simulink model "MOSSE_HDL_code_gen_final"  (Simulink 8.2)
settings: Solver=FixedStepDiscrete  SolverMode=SingleTasking  StartTime=0.0  StopTime=20*640*360  RelTol=1e-3
InitFcn:
  | %% DSPBuilder Start
  | alt_dspbuilder_update_model(bdroot)
  | %% DSPBuilder End
  | param
StopFcn:
  | % r = rcount.Data(:,:);
  | % w = wcount.Data(:,:);
  | % d = dout.Data(:,:);
  | % ir = read.Data(:,:);
  | % iw = write.Data(:,:);
  | % z = double([ir iw d r w]');
  | %logic_analyzer
values from neighbouring files (symbols this model uses):
  Gau = [4035 -3983 3832 -3589 3269 -2890 2472 -2039 1612 -1211 854 -553 ... (4096 elements, 1x4096)]    [Gauss_coeff.mat]    (also in param.m = reshape(conj(Gau'), 1, 4096))
undefined symbols (not defined in the file or in its folder): jet, psr, source_1, source_2, State_Machine, State_Transition_Table1, window_hann
libraries: allblocks_alteradspbuilder2 x182, hdldemolib x2, dspsigattribs x2, dspmtrx3 x2, visionsinks x1, visiontextngfix x1, dspvision x1
(part 2 of 3)

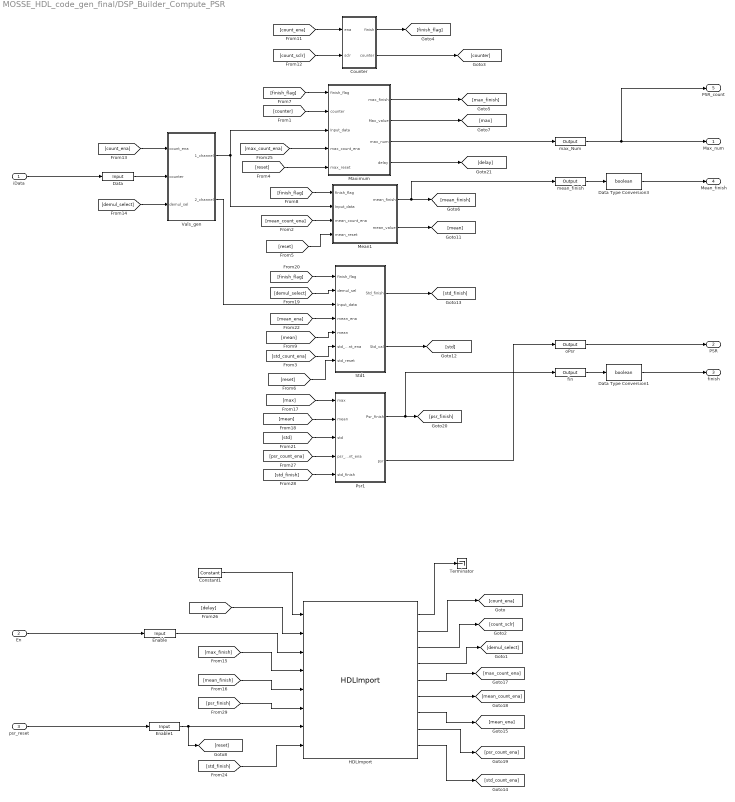
== system MOSSE_HDL_code_gen_final/DSP_Builder_Compute_PSR ==
  iData : Inport
  En : Inport  Port=2
  psr_reset : Inport  Port=3
  Constant1 : allblocks_alteradspbuilder2/Constant  mask_cst=1  BusType=Single Bit  bwl=8  bwr=0  roundMode=Truncate  satMode=Wrap  SpecifyClock=off  allowFloatingPointOverride=on  logOutputs=off  logFile=d:\Project\AutoTracking\model\MOSSE_work\MOSSE_model\MOSSE_Final_models\tb_MOSSE_HDL_final\MOSSE%5FHDL%5Ffinal_DSP%5FBuilder%5FCompute%5FPSR_Constant1.fixedpointlog
  Counter : Subsystem
  Data : allblocks_alteradspbuilder2/Input  iofile=d:\Project\AutoTracking\model\MOSSE_work\MOSSE_model\MOSSE_Final_models\tb_MOSSE_HDL_final\MOSSE%5FHDL%5Ffinal_DSP%5FBuilder%5FCompute%5FPSR_Data.salt  BusType=Signed Integer  bwl=16  bwr=0  SpecifyClock=off  PORTTYPE=Input  externalType=Inferred  allowFloatingPointOverride=on  logOutputs=off
  Data Type Conversion1 : DataTypeConversion  OutDataTypeStr=boolean
  Data Type Conversion3 : DataTypeConversion  OutDataTypeStr=boolean
  Enable : allblocks_alteradspbuilder2/Input  iofile=d:\Project\AutoTracking\model\MOSSE_work\MOSSE_model\MOSSE_Final_models\tb_MOSSE_HDL_final\MOSSE%5FHDL%5Ffinal_DSP%5FBuilder%5FCompute%5FPSR_Enable.salt  BusType=Single Bit  bwl=16  bwr=0  SpecifyClock=off  PORTTYPE=Input  externalType=Inferred  allowFloatingPointOverride=on  logOutputs=off
  Enable1 : allblocks_alteradspbuilder2/Input  iofile=d:\Project\AutoTracking\model\MOSSE_work\MOSSE_model\MOSSE_Final_models\tb_MOSSE_HDL_final\MOSSE%5FHDL%5Ffinal_DSP%5FBuilder%5FCompute%5FPSR_Enable1.salt  BusType=Single Bit  bwl=16  bwr=0  SpecifyClock=off  PORTTYPE=Input  externalType=Inferred  allowFloatingPointOverride=on  logOutputs=off
  HDLImport : allblocks_alteradspbuilder2/HDLImport  entityName=State_Machine_import  inNames=clk_enable delay enable_in max_finish mean_finish psr_finish reset std_finish  inBwls=1 1 1 1 1 1 1 1  inBwrs="0  0  0  0  0  0  0  0"  inTypes=b b b b b b b b  inDelayed="0  0  0  0  0  0  0  0"  outNames=ce_out count_ena count_sclr demul_select max_count_ena mean_count_ena mean_ena psr_count_ena std_count_ena  outBwls=1 1 1 1 1 1 1 1 1  outBwrs="0  0  0  0  0  0  0  0  0"  outTypes=b b b b b b b b b  xmlmapfile=C:\altera\13.0\quartus\dsp_builder\lib\SimgenCMap.xml  vofile=DSPBuilder_MOSSE_HDL_final_import\State_Machine.vo  src_file=psr\State_Machine.v;psr\State_Transition_Table1.v;  TopLevelName=State_Machine  UseQPF=0  n_input_port=8  n_output_port=9  array_clocks=clk  use_systemC_model=off  is_megacore=off  use_dynamic_feedthrough_data=off  use_alphabetical_port_ordering=on  allowFloatingPointOverride=off
  Maximum : Subsystem
  Mean1 : Subsystem
  Psr1 : Subsystem
  Std1 : Subsystem
  Terminator : Terminator
  Vals_gen : Subsystem
  fin : allblocks_alteradspbuilder2/Output  iofile=d:\Project\AutoTracking\model\MOSSE_work\MOSSE_model\MOSSE_Final_models\tb_MOSSE_HDL_final\MOSSE%5FHDL%5Ffinal_DSP%5FBuilder%5FCompute%5FPSR_fin.capture  BusType=Single Bit  bwl=32  bwr=0  externalType=Simulink Fixed Point Type  PORTTYPE=Output  allowFloatingPointOverride=on  logOutputs=off
  max_Num : allblocks_alteradspbuilder2/Output  iofile=d:\Project\AutoTracking\model\MOSSE_work\MOSSE_model\MOSSE_Final_models\tb_MOSSE_HDL_final\MOSSE%5FHDL%5Ffinal_DSP%5FBuilder%5FCompute%5FPSR_max%5FNum.capture  BusType=Signed Integer  bwl=16  bwr=0  externalType=Simulink Fixed Point Type  PORTTYPE=Output  allowFloatingPointOverride=on  logOutputs=off
  mean_finish : allblocks_alteradspbuilder2/Output  iofile=d:\Project\AutoTracking\model\MOSSE_work\MOSSE_model\MOSSE_Final_models\tb_MOSSE_HDL_final\MOSSE%5FHDL%5Ffinal_DSP%5FBuilder%5FCompute%5FPSR_mean%5Ffinish.capture  BusType=Single Bit  bwl=16  bwr=0  externalType=Simulink Fixed Point Type  PORTTYPE=Output  allowFloatingPointOverride=on  logOutputs=off
  oPsr : allblocks_alteradspbuilder2/Output  iofile=d:\Project\AutoTracking\model\MOSSE_work\MOSSE_model\MOSSE_Final_models\tb_MOSSE_HDL_final\MOSSE%5FHDL%5Ffinal_DSP%5FBuilder%5FCompute%5FPSR_oPsr.capture  BusType=Signed Integer  bwl=32  bwr=0  externalType=Simulink Fixed Point Type  PORTTYPE=Output  allowFloatingPointOverride=on  logOutputs=off
  Max_num : Outport
  PSR : Outport  Port=2
  finish : Outport  Port=3
  Mean_finish : Outport  Port=4
  PSR_count : Outport  Port=5
  wires:
  [demul_select] -> Std1/2(demul_sel)
  Data/1 -> Vals_gen/2(counter)
  [demul_select] -> Vals_gen/3(demul_sel)
  Vals_gen/2(2_channel) -> Std1/3(Input_data)
  [finish_flag] -> Std1/1(finish_flag)
  Std1/1(Std_finish) -> [std_finish]
  Mean1/2(mean_value) -> [mean]
  max_Num/1 -> PSR_count/1, Max_num/1
  Maximum/2(Max_value) -> [max]
  [mean] -> Std1/5(mean)
  [mean_ena] -> Std1/4(mean_ena)
  [max] -> Psr1/1(max)
  Maximum/4(delay) -> [delay]
  HDLImport/1 -> Terminator/1
  Constant1/1 -> HDLImport/1
  [psr_finish] -> HDLImport/6
  [std_finish] -> HDLImport/8
  [mean_finish] -> HDLImport/5
  [max_finish] -> HDLImport/4
  [delay] -> HDLImport/2
  Mean1/1(mean_finish) -> mean_finish/1, [mean_finish]
  oPsr/1 -> PSR/1
  [count_ena] -> Vals_gen/1(count_ena)
  Psr1/1(Psr_finish) -> fin/1, [psr_finish]
  Vals_gen/1(1_channel) -> Maximum/3(Input_data), Mean1/2(Input_data)
  [mean_count_ena] -> Mean1/3(mean_count_ena)
  Counter/1(finish) -> [finish_flag]
  Maximum/1(max_finish) -> [max_finish]
  [counter] -> Maximum/2(counter)
  [finish_flag] -> Maximum/1(finish_flag)
  [finish_flag] -> Mean1/1(finish_flag)
  [count_ena] -> Counter/1(ena)
  [count_sclr] -> Counter/2(sclr)
  [std_finish] -> Psr1/5(std_finish)
  Psr1/2(psr) -> oPsr/1
  [mean] -> Psr1/2(mean)
  [std] -> Psr1/3(std)
  Std1/2(Std_val) -> [std]
  [std_count_ena] -> Std1/6(std_count_ena)
  [psr_count_ena] -> Psr1/4(psr_count_ena)
  [max_count_ena] -> Maximum/4(max_count_ena)
  HDLImport/3 -> [count_sclr]
  HDLImport/2 -> [count_ena]
  HDLImport/6 -> [mean_count_ena]
  Enable/1 -> HDLImport/3
  HDLImport/4 -> [demul_select]
  HDLImport/5 -> [max_count_ena]
  HDLImport/7 -> [mean_ena]
  HDLImport/8 -> [psr_count_ena]
  HDLImport/9 -> [std_count_ena]
  Counter/2(counter) -> [counter]
  En/1 -> Enable/1
  iData/1 -> Data/1
  psr_reset/1 -> Enable1/1
  Enable1/1 -> [reset], HDLImport/7
  mean_finish/1 -> Data Type Conversion3/1
  fin/1 -> Data Type Conversion1/1
  Data Type Conversion1/1 -> finish/1
  Data Type Conversion3/1 -> Mean_finish/1
  [reset] -> Maximum/5(max_reset)
  [reset] -> Mean1/4(mean_reset)
  [reset] -> Std1/7(std_reset)
  Maximum/3(max_num) -> max_Num/1

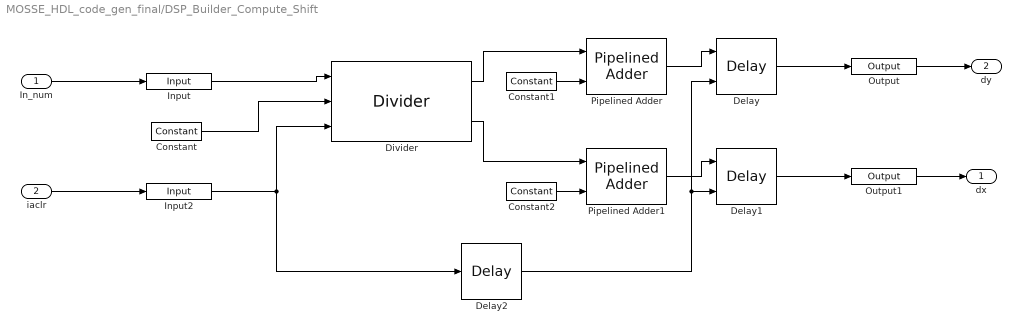
== system MOSSE_HDL_code_gen_final/DSP_Builder_Compute_Shift ==
  In_num : Inport
  iaclr : Inport  Port=2
  Constant : allblocks_alteradspbuilder2/Constant  mask_cst=64  BusType=Unsigned Integer  bwl=8  bwr=0  roundMode=Truncate  satMode=Wrap  SpecifyClock=off  allowFloatingPointOverride=on  logOutputs=off  logFile=C:\Workspace\Autotracking\MOSSE_model\tb_MOSSE_HDL_final\MOSSE%5FHDL%5Ffinal_DSP%5FBuilder%5FCompute%5FShift_Constant.fixedpointlog
  Constant1 : allblocks_alteradspbuilder2/Constant  mask_cst=31  BusType=Signed Integer  bwl=8  bwr=0  roundMode=Truncate  satMode=Wrap  SpecifyClock=off  allowFloatingPointOverride=on  logOutputs=off  logFile=C:\Workspace\Autotracking\MOSSE_model\tb_MOSSE_HDL_final\MOSSE%5FHDL%5Ffinal_DSP%5FBuilder%5FCompute%5FShift_Constant1.fixedpointlog
  Constant2 : allblocks_alteradspbuilder2/Constant  mask_cst=32  BusType=Signed Integer  bwl=8  bwr=0  roundMode=Truncate  satMode=Wrap  SpecifyClock=off  allowFloatingPointOverride=on  logOutputs=off  logFile=C:\Workspace\Autotracking\MOSSE_model\tb_MOSSE_HDL_final\MOSSE%5FHDL%5Ffinal_DSP%5FBuilder%5FCompute%5FShift_Constant2.fixedpointlog
  Delay : allblocks_alteradspbuilder2/Delay  pipeline=1  pipeline_display=1  ClockPhase=1  use_ena=off  use_sclr=on  allowFloatingPointOverride=on  logOutputs=off  logFile=C:\Workspace\Autotracking\MOSSE_model\tb_MOSSE_HDL_final\MOSSE%5FHDL%5Ffinal_DSP%5FBuilder%5FCompute%5FShift_Delay.fixedpointlog  use_init=off  reset_value=1
  Delay1 : allblocks_alteradspbuilder2/Delay  pipeline=1  pipeline_display=1  ClockPhase=1  use_ena=off  use_sclr=on  allowFloatingPointOverride=on  logOutputs=off  logFile=C:\Workspace\Autotracking\MOSSE_model\tb_MOSSE_HDL_final\MOSSE%5FHDL%5Ffinal_DSP%5FBuilder%5FCompute%5FShift_Delay1.fixedpointlog  use_init=off  reset_value=1
  Delay2 : allblocks_alteradspbuilder2/Delay  pipeline=1  pipeline_display=1  ClockPhase=1  use_ena=off  use_sclr=off  allowFloatingPointOverride=on  logOutputs=off  logFile=C:\Workspace\Autotracking\MOSSE_model\tb_MOSSE_HDL_final\MOSSE%5FHDL%5Ffinal_DSP%5FBuilder%5FCompute%5FShift_Delay2.fixedpointlog  use_init=off  reset_value=1
  Divider : allblocks_alteradspbuilder2/Divider  BusType=Unsigned Integer  bwl=12  bwr=0  pipeline=1  pipeline_display=1  use_ena=off  use_aclr=on
  Input : allblocks_alteradspbuilder2/Input  iofile=C:\Workspace\Autotracking\MOSSE_model\tb_MOSSE_HDL_final\MOSSE%5FHDL%5Ffinal_DSP%5FBuilder%5FCompute%5FShift_Input.salt  BusType=Unsigned Integer  bwl=12  bwr=0  SpecifyClock=off  PORTTYPE=Input  externalType=Inferred  allowFloatingPointOverride=on  logOutputs=off
  Input2 : allblocks_alteradspbuilder2/Input  iofile=C:\Workspace\Autotracking\MOSSE_model\tb_MOSSE_HDL_final\MOSSE%5FHDL%5Ffinal_DSP%5FBuilder%5FCompute%5FShift_Input2.salt  BusType=Single Bit  bwl=12  bwr=0  SpecifyClock=off  PORTTYPE=Input  externalType=Inferred  allowFloatingPointOverride=on  logOutputs=off
  Output : allblocks_alteradspbuilder2/Output  iofile=C:\Workspace\Autotracking\MOSSE_model\tb_MOSSE_HDL_final\MOSSE%5FHDL%5Ffinal_DSP%5FBuilder%5FCompute%5FShift_Output.capture  BusType=Signed Integer  bwl=8  bwr=0  externalType=Simulink Fixed Point Type  PORTTYPE=Output  allowFloatingPointOverride=on  logOutputs=off
  Output1 : allblocks_alteradspbuilder2/Output  iofile=C:\Workspace\Autotracking\MOSSE_model\tb_MOSSE_HDL_final\MOSSE%5FHDL%5Ffinal_DSP%5FBuilder%5FCompute%5FShift_Output1.capture  BusType=Signed Integer  bwl=8  bwr=0  externalType=Simulink Fixed Point Type  PORTTYPE=Output  allowFloatingPointOverride=on  logOutputs=off
  Pipelined Adder : allblocks_alteradspbuilder2/Pipelined Adder  BusType=Signed Integer  bwl=12  bwr=0  pipeline=0  pipeline_display=0  AddSubDirection=SUB  use_cin=off  use_ovl=off  use_addsub=off  use_ena=off  use_aclr=off  or_aclr_inputs=on
  Pipelined Adder1 : allblocks_alteradspbuilder2/Pipelined Adder  BusType=Signed Integer  bwl=12  bwr=0  pipeline=0  pipeline_display=0  AddSubDirection=SUB  use_cin=off  use_ovl=off  use_addsub=off  use_ena=off  use_aclr=off  or_aclr_inputs=on
  dx : Outport
  dy : Outport  Port=2
  wires:
  Input/1 -> Divider/1
  Constant/1 -> Divider/2
  In_num/1 -> Input/1
  Output1/1 -> dx/1
  Output/1 -> dy/1
  Divider/1 -> Pipelined Adder/1
  Constant2/1 -> Pipelined Adder1/2
  Pipelined Adder/1 -> Delay/1
  Delay/1 -> Output/1
  Pipelined Adder1/1 -> Delay1/1
  Delay1/1 -> Output1/1
  Divider/2 -> Pipelined Adder1/1
  iaclr/1 -> Input2/1
  Input2/1 -> Delay2/1, Divider/3
  Constant1/1 -> Pipelined Adder/2
  Delay2/1 -> Delay/2, Delay1/2

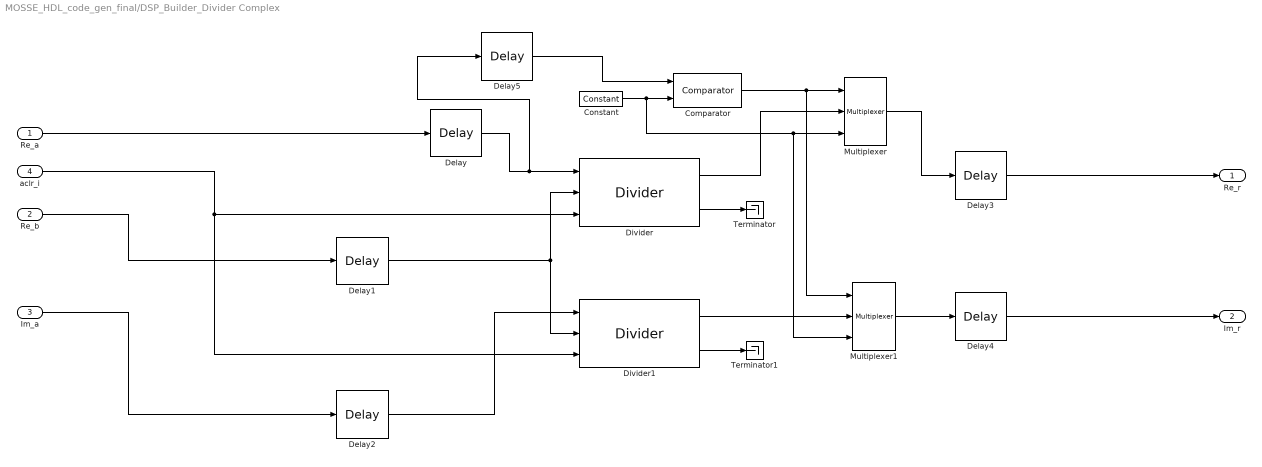
== system MOSSE_HDL_code_gen_final/DSP_Builder_Divider Complex ==
  Re_a : Inport
  Re_b : Inport  Port=2
  Im_a : Inport  Port=3
  aclr_i : Inport  Port=4
  Comparator : allblocks_alteradspbuilder2/Comparator  direction=a == b  pipeline_display=0  allowFloatingPointOverride=on  logOutputs=off  logFile=E:\Project\AutoTracking\model\MOSSE_work\MOSSE_model\test\tb_MOSSE_HDL_code_gen_final\MOSSE%5FHDL%5Fcode%5Fgen%5Ffinal_DSP%5FBuilder%5FDivider+Complex_Comparator.fixedpointlog
  Constant : allblocks_alteradspbuilder2/Constant  mask_cst=0  BusType=Signed Integer  bwl=32  bwr=0  roundMode=Truncate  satMode=Wrap  SpecifyClock=off  allowFloatingPointOverride=on  logOutputs=off  logFile=E:\Project\AutoTracking\model\MOSSE_work\MOSSE_model\test\tb_MOSSE_HDL_code_gen_final\MOSSE%5FHDL%5Fcode%5Fgen%5Ffinal_DSP%5FBuilder%5FDivider+Complex_Constant.fixedpointlog
  Delay : allblocks_alteradspbuilder2/Delay  pipeline=1  pipeline_display=1  ClockPhase=1  use_ena=off  use_sclr=off  allowFloatingPointOverride=on  logOutputs=off  logFile=E:\Project\AutoTracking\model\MOSSE_work\MOSSE_model\test\tb_MOSSE_HDL_code_gen_final\MOSSE%5FHDL%5Fcode%5Fgen%5Ffinal_DSP%5FBuilder%5FDivider+Complex_Delay.fixedpointlog  use_init=off  reset_value=1
  Delay1 : allblocks_alteradspbuilder2/Delay  pipeline=1  pipeline_display=1  ClockPhase=1  use_ena=off  use_sclr=off  allowFloatingPointOverride=on  logOutputs=off  logFile=E:\Project\AutoTracking\model\MOSSE_work\MOSSE_model\test\tb_MOSSE_HDL_code_gen_final\MOSSE%5FHDL%5Fcode%5Fgen%5Ffinal_DSP%5FBuilder%5FDivider+Complex_Delay1.fixedpointlog  use_init=off  reset_value=1
  Delay2 : allblocks_alteradspbuilder2/Delay  pipeline=1  pipeline_display=1  ClockPhase=1  use_ena=off  use_sclr=off  allowFloatingPointOverride=on  logOutputs=off  logFile=E:\Project\AutoTracking\model\MOSSE_work\MOSSE_model\test\tb_MOSSE_HDL_code_gen_final\MOSSE%5FHDL%5Fcode%5Fgen%5Ffinal_DSP%5FBuilder%5FDivider+Complex_Delay2.fixedpointlog  use_init=off  reset_value=1
  Delay3 : allblocks_alteradspbuilder2/Delay  pipeline=1  pipeline_display=1  ClockPhase=1  use_ena=off  use_sclr=off  allowFloatingPointOverride=on  logOutputs=off  logFile=E:\Project\AutoTracking\model\MOSSE_work\MOSSE_model\test\tb_MOSSE_HDL_code_gen_final\MOSSE%5FHDL%5Fcode%5Fgen%5Ffinal_DSP%5FBuilder%5FDivider+Complex_Delay3.fixedpointlog  use_init=off  reset_value=1
  Delay4 : allblocks_alteradspbuilder2/Delay  pipeline=1  pipeline_display=1  ClockPhase=1  use_ena=off  use_sclr=off  allowFloatingPointOverride=on  logOutputs=off  logFile=E:\Project\AutoTracking\model\MOSSE_work\MOSSE_model\test\tb_MOSSE_HDL_code_gen_final\MOSSE%5FHDL%5Fcode%5Fgen%5Ffinal_DSP%5FBuilder%5FDivider+Complex_Delay4.fixedpointlog  use_init=off  reset_value=1
  Delay5 : allblocks_alteradspbuilder2/Delay  pipeline=4  pipeline_display=4  ClockPhase=1  use_ena=off  use_sclr=off  allowFloatingPointOverride=on  logOutputs=off  logFile=E:\Project\AutoTracking\model\MOSSE_work\MOSSE_model\test\tb_MOSSE_HDL_code_gen_final\MOSSE%5FHDL%5Fcode%5Fgen%5Ffinal_DSP%5FBuilder%5FDivider+Complex_Delay5.fixedpointlog  use_init=off  reset_value=1
  Divider : allblocks_alteradspbuilder2/Divider  BusType=Signed Integer  bwl=32  bwr=0  pipeline=4  pipeline_display=4  use_ena=off  use_aclr=on
  Divider1 : allblocks_alteradspbuilder2/Divider  BusType=Signed Integer  bwl=32  bwr=0  pipeline=4  pipeline_display=4  use_ena=off  use_aclr=on
  Multiplexer : allblocks_alteradspbuilder2/Multiplexer  numInputs=2  pipeline=0  oneHot=off  pipeline_display=0  use_ena=off  use_aclr=off  allowFloatingPointOverride=on  logOutputs=off  logFile=E:\Project\AutoTracking\model\MOSSE_work\MOSSE_model\test\tb_MOSSE_HDL_code_gen_final\MOSSE%5FHDL%5Fcode%5Fgen%5Ffinal_DSP%5FBuilder%5FDivider+Complex_Multiplexer.fixedpointlog
  Multiplexer1 : allblocks_alteradspbuilder2/Multiplexer  numInputs=2  pipeline=0  oneHot=off  pipeline_display=0  use_ena=off  use_aclr=off  allowFloatingPointOverride=on  logOutputs=off  logFile=E:\Project\AutoTracking\model\MOSSE_work\MOSSE_model\test\tb_MOSSE_HDL_code_gen_final\MOSSE%5FHDL%5Fcode%5Fgen%5Ffinal_DSP%5FBuilder%5FDivider+Complex_Multiplexer1.fixedpointlog
  Terminator : Terminator
  Terminator1 : Terminator
  Re_r : Outport
  Im_r : Outport  Port=2
  wires:
  Delay3/1 -> Re_r/1
  Divider1/2 -> Terminator1/1
  Divider/2 -> Terminator/1
  Delay4/1 -> Im_r/1
  aclr_i/1 -> Divider/3, Divider1/3
  Re_a/1 -> Delay/1
  Delay1/1 -> Divider1/2, Divider/2
  Re_b/1 -> Delay1/1
  Delay2/1 -> Divider1/1
  Im_a/1 -> Delay2/1
  Divider/1 -> Multiplexer/2
  Multiplexer/1 -> Delay3/1
  Comparator/1 -> Multiplexer1/1, Multiplexer/1
  Constant/1 -> Comparator/2, Multiplexer1/3, Multiplexer/3
  Delay/1 -> Delay5/1, Divider/1
  Delay5/1 -> Comparator/1
  Multiplexer1/1 -> Delay4/1
  Divider1/1 -> Multiplexer1/2

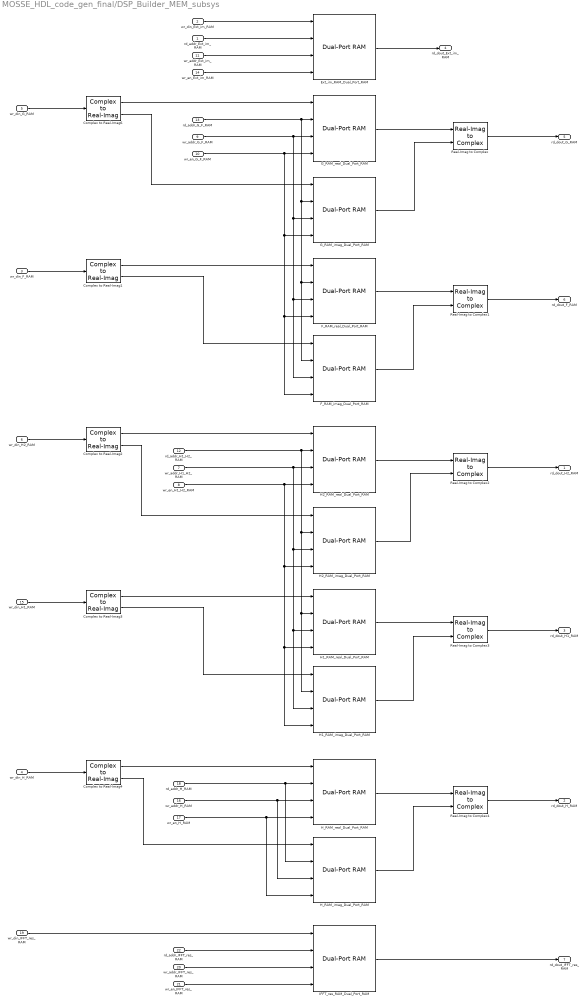
== system MOSSE_HDL_code_gen_final/DSP_Builder_MEM_subsys ==
  rd_addr_Ext_im_RAM : Inport
  wr_din_Ext_im_RAM : Inport  Port=2
  wr_din_F_RAM : Inport  Port=3
  wr_din_H_RAM : Inport  Port=4
  wr_din_G_RAM : Inport  Port=5
  wr_din_H2_RAM : Inport  Port=6
  wr_addr_H1_H2_RAM : Inport  Port=7
  wr_en_H1_H2_RAM : Inport  Port=8
  wr_addr_G_F_RAM : Inport  Port=9
  wr_en_G_F_RAM : Inport  Port=10
  wr_addr_Ext_im_RAM : Inport  Port=11
  rd_addr_H1_H2_RAM : Inport  Port=12
  rd_addr_G_F_RAM : Inport  Port=13
  wr_en_Ext_im_RAM : Inport  Port=14
  wr_din_H1_RAM : Inport  Port=15
  wr_addr_H_RAM : Inport  Port=16
  wr_en_H_RAM : Inport  Port=17
  rd_addr_H_RAM : Inport  Port=18
  wr_din_IFFT_res_RAM : Inport  Port=19
  wr_addr_IFFT_res_RAM : Inport  Port=20
  wr_en_IFFT_res_RAM : Inport  Port=21
  rd_addr_IFFT_res_RAM : Inport  Port=22
  Complex to Real-Imag1 : allblocks_alteradspbuilder2/Complex to Real-Imag  BusType=Signed Integer  bwl=32  bwr=0  pipeline_display=0  allowFloatingPointOverride=on  logOutputs=off  logFile=E:\Project\AutoTracking\model\MOSSE_work\MOSSE_model\test\tb_MOSSE_HDL_code_gen_final\MOSSE%5FHDL%5Fcode%5Fgen%5Ffinal_DSP%5FBuilder%5FMEM%5Fsubsys_Complex+to+Real-Imag1%3A%3Aoutput%5Freal.fixedpointlog,E:\Project\AutoTracking\model\MOSSE_work\MOSSE_model\test\tb_MOSSE_HDL_code_gen_final\MOSSE%5FHDL%5Fcode%5Fgen%5Ffinal_DSP%5FBuilder%5FMEM%5Fsubsys_Complex+to+Real-Imag1%3A%3Aoutput%5Fimag.fixedpointlog,
  Complex to Real-Imag2 : allblocks_alteradspbuilder2/Complex to Real-Imag  BusType=Signed Integer  bwl=32  bwr=0  pipeline_display=0  allowFloatingPointOverride=on  logOutputs=off  logFile=E:\Project\AutoTracking\model\MOSSE_work\MOSSE_model\test\tb_MOSSE_HDL_code_gen_final\MOSSE%5FHDL%5Fcode%5Fgen%5Ffinal_DSP%5FBuilder%5FMEM%5Fsubsys_Complex+to+Real-Imag2%3A%3Aoutput%5Freal.fixedpointlog,E:\Project\AutoTracking\model\MOSSE_work\MOSSE_model\test\tb_MOSSE_HDL_code_gen_final\MOSSE%5FHDL%5Fcode%5Fgen%5Ffinal_DSP%5FBuilder%5FMEM%5Fsubsys_Complex+to+Real-Imag2%3A%3Aoutput%5Fimag.fixedpointlog,
  Complex to Real-Imag3 : allblocks_alteradspbuilder2/Complex to Real-Imag  BusType=Signed Integer  bwl=32  bwr=0  pipeline_display=0  allowFloatingPointOverride=on  logOutputs=off  logFile=E:\Project\AutoTracking\model\MOSSE_work\MOSSE_model\test\tb_MOSSE_HDL_code_gen_final\MOSSE%5FHDL%5Fcode%5Fgen%5Ffinal_DSP%5FBuilder%5FMEM%5Fsubsys_Complex+to+Real-Imag3%3A%3Aoutput%5Freal.fixedpointlog,E:\Project\AutoTracking\model\MOSSE_work\MOSSE_model\test\tb_MOSSE_HDL_code_gen_final\MOSSE%5FHDL%5Fcode%5Fgen%5Ffinal_DSP%5FBuilder%5FMEM%5Fsubsys_Complex+to+Real-Imag3%3A%3Aoutput%5Fimag.fixedpointlog,
  Complex to Real-Imag4 : allblocks_alteradspbuilder2/Complex to Real-Imag  BusType=Signed Integer  bwl=32  bwr=0  pipeline_display=0  allowFloatingPointOverride=on  logOutputs=off  logFile=E:\Project\AutoTracking\model\MOSSE_work\MOSSE_model\test\tb_MOSSE_HDL_code_gen_final\MOSSE%5FHDL%5Fcode%5Fgen%5Ffinal_DSP%5FBuilder%5FMEM%5Fsubsys_Complex+to+Real-Imag4%3A%3Aoutput%5Freal.fixedpointlog,E:\Project\AutoTracking\model\MOSSE_work\MOSSE_model\test\tb_MOSSE_HDL_code_gen_final\MOSSE%5FHDL%5Fcode%5Fgen%5Ffinal_DSP%5FBuilder%5FMEM%5Fsubsys_Complex+to+Real-Imag4%3A%3Aoutput%5Fimag.fixedpointlog,
  Complex to Real-Imag6 : allblocks_alteradspbuilder2/Complex to Real-Imag  BusType=Signed Integer  bwl=32  bwr=0  pipeline_display=0  allowFloatingPointOverride=on  logOutputs=off  logFile=E:\Project\AutoTracking\model\MOSSE_work\MOSSE_model\test\tb_MOSSE_HDL_code_gen_final\MOSSE%5FHDL%5Fcode%5Fgen%5Ffinal_DSP%5FBuilder%5FMEM%5Fsubsys_Complex+to+Real-Imag6%3A%3Aoutput%5Freal.fixedpointlog,E:\Project\AutoTracking\model\MOSSE_work\MOSSE_model\test\tb_MOSSE_HDL_code_gen_final\MOSSE%5FHDL%5Fcode%5Fgen%5Ffinal_DSP%5FBuilder%5FMEM%5Fsubsys_Complex+to+Real-Imag6%3A%3Aoutput%5Fimag.fixedpointlog,
  Ext_im_RAM_Dual_Port_RAM : allblocks_alteradspbuilder2/Dual-Port RAM  numwords=16384  BusType=Unsigned Integer  bwl=8  bwr=0  memory_type=AUTO  ram_type=DualRAM  dont_care=off  initialization=From MATLAB array  init_file=input.hex  init_array=zeros(1,16384)  register_outputs=off  use_ena=off  ClockPhase=1  allowFloatingPointOverride=on  logOutputs=off  logFile=E:\Project\AutoTracking\model\MOSSE_work\MOSSE_model\test\tb_MOSSE_HDL_code_gen_final\MOSSE%5FHDL%5Fcode%5Fgen%5Ffinal_DSP%5FBuilder%5FMEM%5Fsubsys_Ext%5Fim%5FRAM%5FDual%5FPort%5FRAM.fixedpointlog  pipeline_display=1
  F_RAM_imag_Dual_Port_RAM : allblocks_alteradspbuilder2/Dual-Port RAM  numwords=4096  BusType=Signed Integer  bwl=32  bwr=0  memory_type=AUTO  ram_type=DualRAM  dont_care=off  initialization=From MATLAB array  init_file=input.hex  init_array=zeros(1,4096)  register_outputs=off  use_ena=off  ClockPhase=1  allowFloatingPointOverride=on  logOutputs=off  logFile=E:\Project\AutoTracking\model\MOSSE_work\MOSSE_model\test\tb_MOSSE_HDL_code_gen_final\MOSSE%5FHDL%5Fcode%5Fgen%5Ffinal_DSP%5FBuilder%5FMEM%5Fsubsys_F%5FRAM%5Fimag%5FDual%5FPort%5FRAM.fixedpointlog  pipeline_display=1
  F_RAM_real_Dual_Port_RAM : allblocks_alteradspbuilder2/Dual-Port RAM  numwords=4096  BusType=Signed Integer  bwl=32  bwr=0  memory_type=AUTO  ram_type=DualRAM  dont_care=off  initialization=From MATLAB array  init_file=input.hex  init_array=zeros(1,4096)  register_outputs=off  use_ena=off  ClockPhase=1  allowFloatingPointOverride=on  logOutputs=off  logFile=E:\Project\AutoTracking\model\MOSSE_work\MOSSE_model\test\tb_MOSSE_HDL_code_gen_final\MOSSE%5FHDL%5Fcode%5Fgen%5Ffinal_DSP%5FBuilder%5FMEM%5Fsubsys_F%5FRAM%5Freal%5FDual%5FPort%5FRAM.fixedpointlog  pipeline_display=1
  G_RAM_imag_Dual_Port_RAM : allblocks_alteradspbuilder2/Dual-Port RAM  numwords=4096  BusType=Signed Integer  bwl=32  bwr=0  memory_type=AUTO  ram_type=DualRAM  dont_care=off  initialization=From MATLAB array  init_file=input.hex  init_array=zeros(1,4096)  register_outputs=off  use_ena=off  ClockPhase=1  allowFloatingPointOverride=on  logOutputs=off  logFile=E:\Project\AutoTracking\model\MOSSE_work\MOSSE_model\test\tb_MOSSE_HDL_code_gen_final\MOSSE%5FHDL%5Fcode%5Fgen%5Ffinal_DSP%5FBuilder%5FMEM%5Fsubsys_G%5FRAM%5Fimag%5FDual%5FPort%5FRAM.fixedpointlog  pipeline_display=1
  G_RAM_real_Dual_Port_RAM : allblocks_alteradspbuilder2/Dual-Port RAM  numwords=4096  BusType=Signed Integer  bwl=32  bwr=0  memory_type=AUTO  ram_type=DualRAM  dont_care=off  initialization=From MATLAB array  init_file=input.hex  init_array=zeros(1,4096)  register_outputs=off  use_ena=off  ClockPhase=1  allowFloatingPointOverride=on  logOutputs=off  logFile=E:\Project\AutoTracking\model\MOSSE_work\MOSSE_model\test\tb_MOSSE_HDL_code_gen_final\MOSSE%5FHDL%5Fcode%5Fgen%5Ffinal_DSP%5FBuilder%5FMEM%5Fsubsys_G%5FRAM%5Freal%5FDual%5FPort%5FRAM.fixedpointlog  pipeline_display=1
  H1_RAM_imag_Dual_Port_RAM : allblocks_alteradspbuilder2/Dual-Port RAM  numwords=4096  BusType=Signed Integer  bwl=32  bwr=0  memory_type=AUTO  ram_type=DualRAM  dont_care=off  initialization=From MATLAB array  init_file=input.hex  init_array=zeros(1,4096)  register_outputs=off  use_ena=off  ClockPhase=1  allowFloatingPointOverride=on  logOutputs=off  logFile=E:\Project\AutoTracking\model\MOSSE_work\MOSSE_model\test\tb_MOSSE_HDL_code_gen_final\MOSSE%5FHDL%5Fcode%5Fgen%5Ffinal_DSP%5FBuilder%5FMEM%5Fsubsys_H1%5FRAM%5Fimag%5FDual%5FPort%5FRAM.fixedpointlog  pipeline_display=1
  H1_RAM_real_Dual_Port_RAM : allblocks_alteradspbuilder2/Dual-Port RAM  numwords=4096  BusType=Signed Integer  bwl=32  bwr=0  memory_type=AUTO  ram_type=DualRAM  dont_care=off  initialization=From MATLAB array  init_file=input.hex  init_array=zeros(1,4096)  register_outputs=off  use_ena=off  ClockPhase=1  allowFloatingPointOverride=on  logOutputs=off  logFile=E:\Project\AutoTracking\model\MOSSE_work\MOSSE_model\test\tb_MOSSE_HDL_code_gen_final\MOSSE%5FHDL%5Fcode%5Fgen%5Ffinal_DSP%5FBuilder%5FMEM%5Fsubsys_H1%5FRAM%5Freal%5FDual%5FPort%5FRAM.fixedpointlog  pipeline_display=1
  H2_RAM_imag_Dual_Port_RAM : allblocks_alteradspbuilder2/Dual-Port RAM  numwords=4096  BusType=Signed Integer  bwl=32  bwr=0  memory_type=AUTO  ram_type=DualRAM  dont_care=off  initialization=From MATLAB array  init_file=input.hex  init_array=zeros(1,4096)  register_outputs=off  use_ena=off  ClockPhase=1  allowFloatingPointOverride=on  logOutputs=off  logFile=E:\Project\AutoTracking\model\MOSSE_work\MOSSE_model\test\tb_MOSSE_HDL_code_gen_final\MOSSE%5FHDL%5Fcode%5Fgen%5Ffinal_DSP%5FBuilder%5FMEM%5Fsubsys_H2%5FRAM%5Fimag%5FDual%5FPort%5FRAM.fixedpointlog  pipeline_display=1
  H2_RAM_real_Dual_Port_RAM : allblocks_alteradspbuilder2/Dual-Port RAM  numwords=4096  BusType=Signed Integer  bwl=32  bwr=0  memory_type=AUTO  ram_type=DualRAM  dont_care=off  initialization=From MATLAB array  init_file=input.hex  init_array=zeros(1,4096)  register_outputs=off  use_ena=off  ClockPhase=1  allowFloatingPointOverride=on  logOutputs=off  logFile=E:\Project\AutoTracking\model\MOSSE_work\MOSSE_model\test\tb_MOSSE_HDL_code_gen_final\MOSSE%5FHDL%5Fcode%5Fgen%5Ffinal_DSP%5FBuilder%5FMEM%5Fsubsys_H2%5FRAM%5Freal%5FDual%5FPort%5FRAM.fixedpointlog  pipeline_display=1
  H_RAM_imag_Dual_Port_RAM : allblocks_alteradspbuilder2/Dual-Port RAM  numwords=4096  BusType=Signed Integer  bwl=32  bwr=0  memory_type=AUTO  ram_type=DualRAM  dont_care=off  initialization=From MATLAB array  init_file=input.hex  init_array=zeros(1,4096)  register_outputs=off  use_ena=off  ClockPhase=1  allowFloatingPointOverride=on  logOutputs=off  logFile=E:\Project\AutoTracking\model\MOSSE_work\MOSSE_model\test\tb_MOSSE_HDL_code_gen_final\MOSSE%5FHDL%5Fcode%5Fgen%5Ffinal_DSP%5FBuilder%5FMEM%5Fsubsys_H%5FRAM%5Fimag%5FDual%5FPort%5FRAM.fixedpointlog  pipeline_display=1
  H_RAM_real_Dual_Port_RAM : allblocks_alteradspbuilder2/Dual-Port RAM  numwords=4096  BusType=Signed Integer  bwl=32  bwr=0  memory_type=AUTO  ram_type=DualRAM  dont_care=off  initialization=From MATLAB array  init_file=input.hex  init_array=zeros(1,4096)  register_outputs=off  use_ena=off  ClockPhase=1  allowFloatingPointOverride=on  logOutputs=off  logFile=E:\Project\AutoTracking\model\MOSSE_work\MOSSE_model\test\tb_MOSSE_HDL_code_gen_final\MOSSE%5FHDL%5Fcode%5Fgen%5Ffinal_DSP%5FBuilder%5FMEM%5Fsubsys_H%5FRAM%5Freal%5FDual%5FPort%5FRAM.fixedpointlog  pipeline_display=1
  IFFT_res_RAM_Dual_Port_RAM : allblocks_alteradspbuilder2/Dual-Port RAM  numwords=4096  BusType=Signed Integer  bwl=16  bwr=0  memory_type=AUTO  ram_type=DualRAM  dont_care=off  initialization=From MATLAB array  init_file=input.hex  init_array=zeros(1,4096)  register_outputs=off  use_ena=off  ClockPhase=1  allowFloatingPointOverride=on  logOutputs=off  logFile=E:\Project\AutoTracking\model\MOSSE_work\MOSSE_model\test\tb_MOSSE_HDL_code_gen_final\MOSSE%5FHDL%5Fcode%5Fgen%5Ffinal_DSP%5FBuilder%5FMEM%5Fsubsys_IFFT%5Fres%5FRAM%5FDual%5FPort%5FRAM.fixedpointlog  pipeline_display=1
  Real-Imag to Complex : allblocks_alteradspbuilder2/Real-Imag to Complex  BusType=Signed Integer  bwl=32  bwr=0  pipeline_display=0  allowFloatingPointOverride=on  logOutputs=off  logFile=E:\Project\AutoTracking\model\MOSSE_work\MOSSE_model\test\tb_MOSSE_HDL_code_gen_final\MOSSE%5FHDL%5Fcode%5Fgen%5Ffinal_DSP%5FBuilder%5FMEM%5Fsubsys_Real-Imag+to+Complex.fixedpointlog
  Real-Imag to Complex1 : allblocks_alteradspbuilder2/Real-Imag to Complex  BusType=Signed Integer  bwl=32  bwr=0  pipeline_display=0  allowFloatingPointOverride=on  logOutputs=off  logFile=E:\Project\AutoTracking\model\MOSSE_work\MOSSE_model\test\tb_MOSSE_HDL_code_gen_final\MOSSE%5FHDL%5Fcode%5Fgen%5Ffinal_DSP%5FBuilder%5FMEM%5Fsubsys_Real-Imag+to+Complex1.fixedpointlog
  Real-Imag to Complex2 : allblocks_alteradspbuilder2/Real-Imag to Complex  BusType=Signed Integer  bwl=32  bwr=0  pipeline_display=0  allowFloatingPointOverride=on  logOutputs=off  logFile=E:\Project\AutoTracking\model\MOSSE_work\MOSSE_model\test\tb_MOSSE_HDL_code_gen_final\MOSSE%5FHDL%5Fcode%5Fgen%5Ffinal_DSP%5FBuilder%5FMEM%5Fsubsys_Real-Imag+to+Complex2.fixedpointlog
  Real-Imag to Complex3 : allblocks_alteradspbuilder2/Real-Imag to Complex  BusType=Signed Integer  bwl=32  bwr=0  pipeline_display=0  allowFloatingPointOverride=on  logOutputs=off  logFile=E:\Project\AutoTracking\model\MOSSE_work\MOSSE_model\test\tb_MOSSE_HDL_code_gen_final\MOSSE%5FHDL%5Fcode%5Fgen%5Ffinal_DSP%5FBuilder%5FMEM%5Fsubsys_Real-Imag+to+Complex3.fixedpointlog
  Real-Imag to Complex4 : allblocks_alteradspbuilder2/Real-Imag to Complex  BusType=Signed Integer  bwl=32  bwr=0  pipeline_display=0  allowFloatingPointOverride=on  logOutputs=off  logFile=E:\Project\AutoTracking\model\MOSSE_work\MOSSE_model\test\tb_MOSSE_HDL_code_gen_final\MOSSE%5FHDL%5Fcode%5Fgen%5Ffinal_DSP%5FBuilder%5FMEM%5Fsubsys_Real-Imag+to+Complex4.fixedpointlog
  rd_dout_H2_RAM : Outport
  rd_dout_H_RAM : Outport  Port=2
  rd_dout_H1_RAM : Outport  Port=3
  rd_dout_Ext_im_RAM : Outport  Port=4
  rd_dout_G_RAM : Outport  Port=5
  rd_dout_F_RAM : Outport  Port=6
  rd_dout_IFFT_res_RAM : Outport  Port=7
  wires:
  wr_din_Ext_im_RAM/1 -> Ext_im_RAM_Dual_Port_RAM/1
  rd_addr_Ext_im_RAM/1 -> Ext_im_RAM_Dual_Port_RAM/2
  wr_addr_Ext_im_RAM/1 -> Ext_im_RAM_Dual_Port_RAM/3
  wr_en_Ext_im_RAM/1 -> Ext_im_RAM_Dual_Port_RAM/4
  Ext_im_RAM_Dual_Port_RAM/1 -> rd_dout_Ext_im_RAM/1
  rd_addr_G_F_RAM/1 -> F_RAM_real_Dual_Port_RAM/2, F_RAM_imag_Dual_Port_RAM/2, G_RAM_imag_Dual_Port_RAM/2, G_RAM_real_Dual_Port_RAM/2
  wr_addr_G_F_RAM/1 -> G_RAM_imag_Dual_Port_RAM/3, F_RAM_real_Dual_Port_RAM/3, F_RAM_imag_Dual_Port_RAM/3, G_RAM_real_Dual_Port_RAM/3
  wr_en_G_F_RAM/1 -> G_RAM_imag_Dual_Port_RAM/4, F_RAM_real_Dual_Port_RAM/4, F_RAM_imag_Dual_Port_RAM/4, G_RAM_real_Dual_Port_RAM/4
  Complex to Real-Imag1/1 -> F_RAM_real_Dual_Port_RAM/1
  F_RAM_real_Dual_Port_RAM/1 -> Real-Imag to Complex1/1
  Complex to Real-Imag1/2 -> F_RAM_imag_Dual_Port_RAM/1
  F_RAM_imag_Dual_Port_RAM/1 -> Real-Imag to Complex1/2
  Complex to Real-Imag2/1 -> H2_RAM_real_Dual_Port_RAM/1
  rd_addr_H1_H2_RAM/1 -> H1_RAM_real_Dual_Port_RAM/2, H1_RAM_imag_Dual_Port_RAM/2, H2_RAM_imag_Dual_Port_RAM/2, H2_RAM_real_Dual_Port_RAM/2
  wr_addr_H1_H2_RAM/1 -> H2_RAM_imag_Dual_Port_RAM/3, H1_RAM_real_Dual_Port_RAM/3, H1_RAM_imag_Dual_Port_RAM/3, H2_RAM_real_Dual_Port_RAM/3
  wr_en_H1_H2_RAM/1 -> H2_RAM_imag_Dual_Port_RAM/4, H1_RAM_real_Dual_Port_RAM/4, H1_RAM_imag_Dual_Port_RAM/4, H2_RAM_real_Dual_Port_RAM/4
  H2_RAM_real_Dual_Port_RAM/1 -> Real-Imag to Complex2/1
  Complex to Real-Imag2/2 -> H2_RAM_imag_Dual_Port_RAM/1
  H2_RAM_imag_Dual_Port_RAM/1 -> Real-Imag to Complex2/2
  Complex to Real-Imag3/1 -> H1_RAM_real_Dual_Port_RAM/1
  H1_RAM_real_Dual_Port_RAM/1 -> Real-Imag to Complex3/1
  Complex to Real-Imag3/2 -> H1_RAM_imag_Dual_Port_RAM/1
  H1_RAM_imag_Dual_Port_RAM/1 -> Real-Imag to Complex3/2
  Complex to Real-Imag4/1 -> H_RAM_real_Dual_Port_RAM/1
  H_RAM_real_Dual_Port_RAM/1 -> Real-Imag to Complex4/1
  Complex to Real-Imag4/2 -> H_RAM_imag_Dual_Port_RAM/1
  H_RAM_imag_Dual_Port_RAM/1 -> Real-Imag to Complex4/2
  rd_addr_H_RAM/1 -> H_RAM_imag_Dual_Port_RAM/2, H_RAM_real_Dual_Port_RAM/2
  wr_en_H_RAM/1 -> H_RAM_imag_Dual_Port_RAM/4, H_RAM_real_Dual_Port_RAM/4
  wr_addr_H_RAM/1 -> H_RAM_imag_Dual_Port_RAM/3, H_RAM_real_Dual_Port_RAM/3
  wr_en_IFFT_res_RAM/1 -> IFFT_res_RAM_Dual_Port_RAM/4
  wr_addr_IFFT_res_RAM/1 -> IFFT_res_RAM_Dual_Port_RAM/3
  rd_addr_IFFT_res_RAM/1 -> IFFT_res_RAM_Dual_Port_RAM/2
  G_RAM_real_Dual_Port_RAM/1 -> Real-Imag to Complex/1
  G_RAM_imag_Dual_Port_RAM/1 -> Real-Imag to Complex/2
  Real-Imag to Complex/1 -> rd_dout_G_RAM/1
  wr_din_F_RAM/1 -> Complex to Real-Imag1/1
  Real-Imag to Complex1/1 -> rd_dout_F_RAM/1
  Real-Imag to Complex2/1 -> rd_dout_H2_RAM/1
  Real-Imag to Complex3/1 -> rd_dout_H1_RAM/1
  Real-Imag to Complex4/1 -> rd_dout_H_RAM/1
  wr_din_H2_RAM/1 -> Complex to Real-Imag2/1
  wr_din_H1_RAM/1 -> Complex to Real-Imag3/1
  wr_din_H_RAM/1 -> Complex to Real-Imag4/1
  Complex to Real-Imag6/1 -> G_RAM_real_Dual_Port_RAM/1
  Complex to Real-Imag6/2 -> G_RAM_imag_Dual_Port_RAM/1
  wr_din_G_RAM/1 -> Complex to Real-Imag6/1
  IFFT_res_RAM_Dual_Port_RAM/1 -> rd_dout_IFFT_res_RAM/1
  wr_din_IFFT_res_RAM/1 -> IFFT_res_RAM_Dual_Port_RAM/1

== system MOSSE_HDL_code_gen_final/DSP_Builder_Mult_complex ==
  F* : Inport
  F : Inport  Port=2
  rst : Inport  Port=3
  enb : Inport  Port=4
  Complex Product : allblocks_alteradspbuilder2/Complex Product  BusType=Inferred  bwl=8  bwr=0  pipeline_register=Multiplier Only  pipeline_display=1  use_ena=off  use_aclr=off  UseDedicatedCircuitry=off  allowFloatingPointOverride=on  logOutputs=off  logFile=E:\Project\AutoTracking\AutoTrack\Model\MOSSE_algorithm\MOSSE_simulink\tb_MOSSE_HDL_code_gen_final\MOSSE%5FHDL%5Fcode%5Fgen%5Ffinal_DSP%5FBuilder%5FMult%5Fcomplex_Complex+Product.fixedpointlog
  Complex Product1 : allblocks_alteradspbuilder2/Complex Product  BusType=Inferred  bwl=8  bwr=0  pipeline_register=Multiplier Only  pipeline_display=1  use_ena=off  use_aclr=off  UseDedicatedCircuitry=off  allowFloatingPointOverride=on  logOutputs=off  logFile=E:\Project\AutoTracking\AutoTrack\Model\MOSSE_algorithm\MOSSE_simulink\tb_MOSSE_HDL_code_gen_final\MOSSE%5FHDL%5Fcode%5Fgen%5Ffinal_DSP%5FBuilder%5FMult%5Fcomplex_Complex+Product1.fixedpointlog
  Gauss_table : Subsystem
  Real-Imag to Complex : allblocks_alteradspbuilder2/Real-Imag to Complex  BusType=Signed Integer  bwl=16  bwr=0  pipeline_display=0  allowFloatingPointOverride=on  logOutputs=off  logFile=E:\Project\AutoTracking\AutoTrack\Model\MOSSE_algorithm\MOSSE_simulink\tb_MOSSE_HDL_code_gen_final\MOSSE%5FHDL%5Fcode%5Fgen%5Ffinal_DSP%5FBuilder%5FMult%5Fcomplex_Real-Imag+to+Complex.fixedpointlog
  H2 : Outport
  H1 : Outport  Port=2
  wires:
  Gauss_table/1(Coeff_real) -> Real-Imag to Complex/1
  Gauss_table/2(Coeff_imag) -> Real-Imag to Complex/2
  Real-Imag to Complex/1 -> Complex Product/1
  rst/1 -> Gauss_table/1(rst)
  enb/1 -> Gauss_table/2(enb)
  F*/1 -> Complex Product1/2, Complex Product/2
  F/1 -> Complex Product1/1
  Complex Product/1 -> H1/1
  Complex Product1/1 -> H2/1

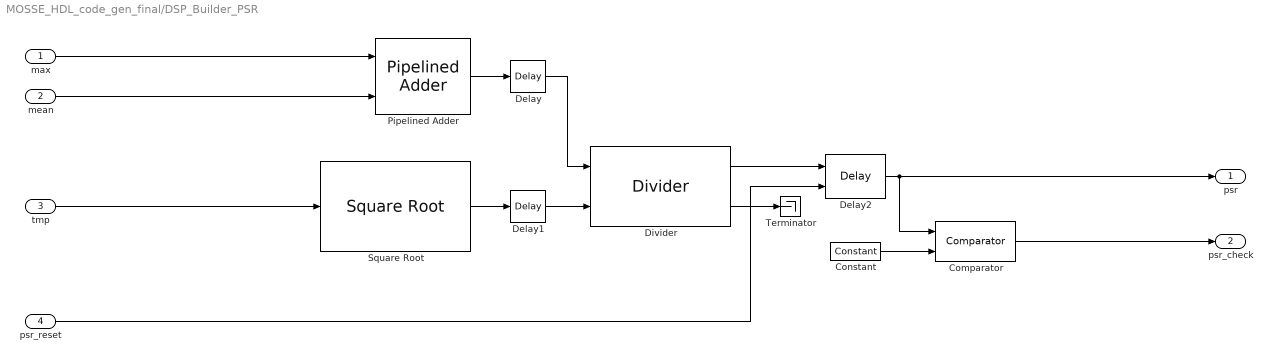
== system MOSSE_HDL_code_gen_final/DSP_Builder_PSR ==
  max : Inport
  mean : Inport  Port=2
  tmp : Inport  Port=3
  psr_reset : Inport  Port=4
  Comparator : allblocks_alteradspbuilder2/Comparator  direction=a > b  pipeline_display=0  allowFloatingPointOverride=on  logOutputs=off  logFile=E:\Project\AutoTracking\model\MOSSE_work\MOSSE_model\test\tb_MOSSE_HDL_code_gen_final\MOSSE%5FHDL%5Fcode%5Fgen%5Ffinal_DSP%5FBuilder%5FPSR_Comparator.fixedpointlog
  Constant : allblocks_alteradspbuilder2/Constant  mask_cst=PSR  BusType=Signed Integer  bwl=16  bwr=0  roundMode=Truncate  satMode=Wrap  SpecifyClock=off  allowFloatingPointOverride=on  logOutputs=off  logFile=E:\Project\AutoTracking\model\MOSSE_work\MOSSE_model\test\tb_MOSSE_HDL_code_gen_final\MOSSE%5FHDL%5Fcode%5Fgen%5Ffinal_DSP%5FBuilder%5FPSR_Constant.fixedpointlog
  Delay : allblocks_alteradspbuilder2/Delay  pipeline=1  pipeline_display=1  ClockPhase=1  use_ena=off  use_sclr=off  allowFloatingPointOverride=on  logOutputs=off  logFile=E:\Project\AutoTracking\model\MOSSE_work\MOSSE_model\test\tb_MOSSE_HDL_code_gen_final\MOSSE%5FHDL%5Fcode%5Fgen%5Ffinal_DSP%5FBuilder%5FPSR_Delay.fixedpointlog  use_init=off  reset_value=1
  Delay1 : allblocks_alteradspbuilder2/Delay  pipeline=1  pipeline_display=1  ClockPhase=1  use_ena=off  use_sclr=off  allowFloatingPointOverride=on  logOutputs=off  logFile=E:\Project\AutoTracking\model\MOSSE_work\MOSSE_model\test\tb_MOSSE_HDL_code_gen_final\MOSSE%5FHDL%5Fcode%5Fgen%5Ffinal_DSP%5FBuilder%5FPSR_Delay1.fixedpointlog  use_init=off  reset_value=1
  Delay2 : allblocks_alteradspbuilder2/Delay  pipeline=1  pipeline_display=1  ClockPhase=1  use_ena=off  use_sclr=on  allowFloatingPointOverride=on  logOutputs=off  logFile=E:\Project\AutoTracking\model\MOSSE_work\MOSSE_model\test\tb_MOSSE_HDL_code_gen_final\MOSSE%5FHDL%5Fcode%5Fgen%5Ffinal_DSP%5FBuilder%5FPSR_Delay2.fixedpointlog  use_init=off  reset_value=1
  Divider : allblocks_alteradspbuilder2/Divider  BusType=Signed Integer  bwl=32  bwr=0  pipeline=5  pipeline_display=5  use_ena=off  use_aclr=off
  Pipelined Adder : allblocks_alteradspbuilder2/Pipelined Adder  BusType=Signed Integer  bwl=32  bwr=0  pipeline=0  pipeline_display=0  AddSubDirection=SUB  use_cin=off  use_ovl=off  use_addsub=off  use_ena=off  use_aclr=off  or_aclr_inputs=on
  Square Root : allblocks_alteradspbuilder2/Square Root  BusType=Unsigned Integer  bwl=44  bwr=0  pipeline=2  pipeline_display=2  use_remain=off  use_ena=off  use_aclr=off
  Terminator : Terminator
  psr : Outport
  psr_check : Outport  Port=2
  wires:
  Pipelined Adder/1 -> Delay/1
  Square Root/1 -> Delay1/1
  Divider/1 -> Delay2/1
  max/1 -> Pipelined Adder/1
  mean/1 -> Pipelined Adder/2
  tmp/1 -> Square Root/1
  Divider/2 -> Terminator/1
  Delay2/1 -> psr/1, Comparator/1
  Delay1/1 -> Divider/2
  Delay/1 -> Divider/1
  psr_reset/1 -> Delay2/2
  Constant/1 -> Comparator/2
  Comparator/1 -> psr_check/1

== system MOSSE_HDL_code_gen_final/DSP_Builder_Smoothing_Window ==
  ipixel : Inport
  rst : Inport  Port=2
  enb : Inport  Port=3
  Barrel Shifter : allblocks_alteradspbuilder2/Barrel Shifter  BusType=Unsigned Integer  bwl=16  bwr=8  pipeline=off  infer_distance=off  distance_length=4  ShiftDirection=Shift right  use_ena=off  use_aclr=off  UseDedicatedCircuitry=off  pipeline_display=0  allowFloatingPointOverride=on  logOutputs=off  logFile=E:\Project\AutoTracking\model\MOSSE_work\MOSSE_model\test\tb_MOSSE_HDL_code_gen_final\MOSSE%5FHDL%5Fcode%5Fgen%5Ffinal_DSP%5FBuilder%5FSmoothing%5FWindow_Barrel+Shifter.fixedpointlog
  Constant : allblocks_alteradspbuilder2/Constant  mask_cst=8  BusType=Unsigned Integer  bwl=4  bwr=0  roundMode=Truncate  satMode=Wrap  SpecifyClock=off  allowFloatingPointOverride=on  logOutputs=off  logFile=E:\Project\AutoTracking\model\MOSSE_work\MOSSE_model\test\tb_MOSSE_HDL_code_gen_final\MOSSE%5FHDL%5Fcode%5Fgen%5Ffinal_DSP%5FBuilder%5FSmoothing%5FWindow_Constant.fixedpointlog
  Counter : allblocks_alteradspbuilder2/Counter  BusType=Unsigned Integer  bwl=12  bwr=0  use_modulo=off  modulo=255  SpecifyClock=off  direction=Increment  use_sload=off  use_sset=off  svalue=1  use_clk_ena=off  use_ena=on  use_sclr=on  pipeline_display=1
  Product : allblocks_alteradspbuilder2/Product  BusType=Unsigned Integer  bwl=8  bwr=0  pipeline=1  pipeline_display=1  phase_selection=1  use_ena=off  use_aclr=off  UseLPM=off  UseDedicatedCircuitry=off  allowFloatingPointOverride=on  logOutputs=off  logFile=E:\Project\AutoTracking\model\MOSSE_work\MOSSE_model\test\tb_MOSSE_HDL_code_gen_final\MOSSE%5FHDL%5Fcode%5Fgen%5Ffinal_DSP%5FBuilder%5FSmoothing%5FWindow_Product.fixedpointlog
  ROM : allblocks_alteradspbuilder2/ROM  numwords=4096  BusType=Unsigned Integer  bwl=8  bwr=0  memory_type=AUTO  ram_type=ROM  initialization=From MATLAB array  init_file=input.hex  init_array=reshape(window_hann', 1, 4096)  register_outputs=off  use_ena=off  ClockPhase=1  pipeline_display=1  allowFloatingPointOverride=on  logOutputs=off  logFile=E:\Project\AutoTracking\model\MOSSE_work\MOSSE_model\test\tb_MOSSE_HDL_code_gen_final\MOSSE%5FHDL%5Fcode%5Fgen%5Ffinal_DSP%5FBuilder%5FSmoothing%5FWindow_ROM.fixedpointlog  enable_runtime_mod=off  instance_name=AAAA
  opixel : Outport
  wires:
  Counter/1 -> ROM/1
  ipixel/1 -> Product/1
  Barrel Shifter/1 -> opixel/1
  enb/1 -> Counter/1
  rst/1 -> Counter/2
  Product/1 -> Barrel Shifter/1
  Constant/1 -> Barrel Shifter/2
  ROM/1 -> Product/2

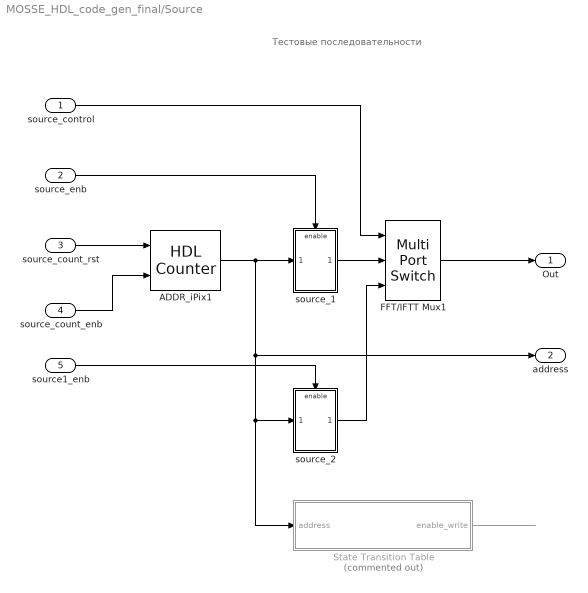
== system MOSSE_HDL_code_gen_final/Source ==
  note: Тестовые последовательности
  source_control : Inport
  source_enb : Inport  Port=2
  source_count_rst : Inport  Port=3
  source_count_enb : Inport  Port=4
  source1_enb : Inport  Port=5
  ADDR_iPix1 : hdldemolib/HDL Counter  CountType=Free running  CountInit=0  CountStep=1  CountMax=100  CountFromType=Initial value  CountFrom=0  CountResetPort=on  CountLoadPort=off  CountEnbPort=on  CountDirPort=off  CountDataType=Unsigned  CountWordLen=32  CountFracLen=0  CountSampTime=1
  FFT/IFTT Mux1 : MultiPortSwitch  DataPortOrder=Zero-based contiguous  Inputs=2  zeroidx=on  OutDataTypeStr=fixdt(1,24,0)  SampleTime=1
  State Transition Table : State Transition Table  Commented=on  TreatAsAtomicUnit=on
  source_1 : Subsystem
  source_2 : Subsystem
  Out : Outport
  address : Outport  Port=2
  wires:
  ADDR_iPix1/1 -> address/1, State Transition Table/1(address), source_2/1(In1), source_1/1(In1)
  source_enb/1 -> source_1/Enable
  source1_enb/1 -> source_2/Enable
  source_count_enb/1 -> ADDR_iPix1/2
  FFT/IFTT Mux1/1 -> Out/1
  source_count_rst/1 -> ADDR_iPix1/1
  source_1/1(Out1) -> FFT/IFTT Mux1/2
  source_control/1 -> FFT/IFTT Mux1/1
  source_2/1(Out1) -> FFT/IFTT Mux1/3
  State Transition Table/1(enable_write) -> ?

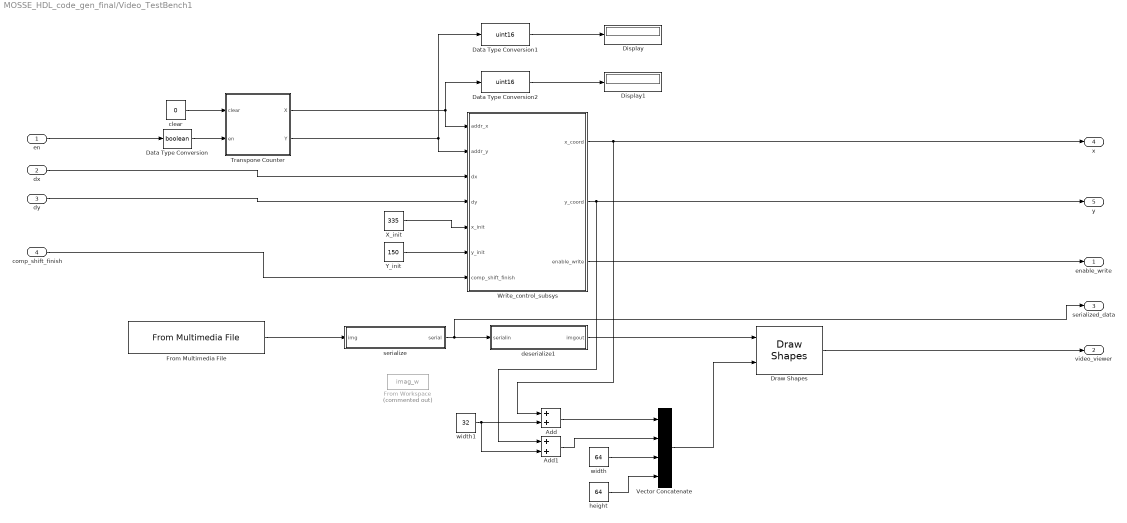
== system MOSSE_HDL_code_gen_final/Video_TestBench1 ==
  en : Inport
  dx : Inport  Port=2
  dy : Inport  Port=3
  comp_shift_finish : Inport  Port=4
  Add : Sum  AccumDataTypeStr=uint16
  Add1 : Sum  AccumDataTypeStr=uint16
  Data Type Conversion : DataTypeConversion  OutDataTypeStr=boolean
  Data Type Conversion1 : DataTypeConversion  OutDataTypeStr=uint16
  Data Type Conversion2 : DataTypeConversion  OutDataTypeStr=uint16
  Display : Display
  Display1 : Display
  Draw Shapes : visiontextngfix/Draw Shapes  shape=Rectangles  fill=off  fillClrSource=Specify via dialog  display=User-specified value  intensity=200  color=[255]  opacity=0.6  viewport=Entire image  antialiasing=off  inType=Obsolete  imagePorts=One multidimensional signal  prodOutputMode=Binary point scaling  prodOutputWordLength=32  prodOutputFracLength=14  memoryMode=Specify word length  memoryWordLength=16  memoryFracLength=15  roundingMode=Floor  overflowMode=off
  From Workspace : FromWorkspace  Commented=on  VariableName=imag_w  SampleTime=1
  From Multimedia File : dspvision/From Multimedia File  inputFilename=E:\Project\AutoTracking\model\MOSSE_work\MOSSE_model\test\klt_algorithm_robustness_640x360.avi  loop=on  numPlays=inf  outputStreams=Video only  videoDataType=uint8  audioDataType=int16  inheritSampleTime=off  userDefinedSampleTime=640*360  noAudioOutput=off  isIntensityVideo=off  fourcc=Intensity  colorVideoFormat=One multidimensional signal  outputEOF=off  dataOrg=Column-major  audioFrameSize=1024  computeAudioFrameSize=off  outSamplingMode=Sample based
  Transpone Counter : MATLAB Function
  Vector Concatenate : Concatenate  NumInputs=4
  Write_control_subsys : Subsystem
  X_init : Constant  Value=335  OutDataTypeStr=uint16
  Y_init : Constant  Value=150  OutDataTypeStr=uint16
  clear : Constant  Value=0  OutDataTypeStr=boolean
  deserialize1 : Subsystem
  height : Constant  Value=64  OutDataTypeStr=uint16
  serialize : Subsystem
  width : Constant  Value=64  OutDataTypeStr=uint16
  width1 : Constant  Value=32  OutDataTypeStr=uint16
  enable_write : Outport
  video_viewer : Outport  Port=2
  serialized_data : Outport  Port=3
  x : Outport  Port=4
  y : Outport  Port=5
  wires:
  From Multimedia File/1 -> serialize/1(img)
  deserialize1/1(imgout) -> Draw Shapes/1
  serialize/1(serial) -> deserialize1/1(serialin), serialized_data/1
  Transpone Counter/2(Y) -> Write_control_subsys/2(addr_y), Data Type Conversion1/1
  Transpone Counter/1(X) -> Write_control_subsys/1(addr_x), Data Type Conversion2/1
  Data Type Conversion/1 -> Transpone Counter/2(en)
  clear/1 -> Transpone Counter/1(clear)
  en/1 -> Data Type Conversion/1
  Draw Shapes/1 -> video_viewer/1
  width/1 -> Vector Concatenate/3
  height/1 -> Vector Concatenate/4
  Vector Concatenate/1 -> Draw Shapes/2
  Add1/1 -> Vector Concatenate/2
  Add/1 -> Vector Concatenate/1
  Data Type Conversion1/1 -> Display/1
  Data Type Conversion2/1 -> Display1/1
  width1/1 -> Add/2, Add1/2
  Write_control_subsys/1(x_coord) -> x/1, Add/1
  Write_control_subsys/2(y_coord) -> y/1, Add1/1
  dx/1 -> Write_control_subsys/3(dx)
  X_init/1 -> Write_control_subsys/5(x_init)
  dy/1 -> Write_control_subsys/4(dy)
  comp_shift_finish/1 -> Write_control_subsys/7(comp_shift_finish)
  Write_control_subsys/3(enable_write) -> enable_write/1
  Y_init/1 -> Write_control_subsys/6(y_init)

== system MOSSE_HDL_code_gen_final/DSP_Builder_Compute_PSR/Counter ==
  ena : Inport
  sclr : Inport  Port=2
  Comparator1 : allblocks_alteradspbuilder2/Comparator  direction=a == b  pipeline_display=0  allowFloatingPointOverride=on  logOutputs=off  logFile=d:\Project\AutoTracking\model\MOSSE_work\MOSSE_model\MOSSE_Final_models\tb_MOSSE_HDL_final\MOSSE%5FHDL%5Ffinal_DSP%5FBuilder%5FCompute%5FPSR_Counter_Comparator1.fixedpointlog
  Constant : allblocks_alteradspbuilder2/Constant  mask_cst=4095  BusType=Unsigned Integer  bwl=16  bwr=0  roundMode=Truncate  satMode=Wrap  SpecifyClock=off  allowFloatingPointOverride=on  logOutputs=off  logFile=d:\Project\AutoTracking\model\MOSSE_work\MOSSE_model\MOSSE_Final_models\tb_MOSSE_HDL_final\MOSSE%5FHDL%5Ffinal_DSP%5FBuilder%5FCompute%5FPSR_Counter_Constant.fixedpointlog
  Counter : allblocks_alteradspbuilder2/Counter  BusType=Unsigned Integer  bwl=16  bwr=0  use_modulo=on  modulo=4100  SpecifyClock=off  direction=Increment  use_sload=off  use_sset=off  svalue=1  use_clk_ena=off  use_ena=on  use_sclr=on  pipeline_display=1
  finish : Outport
  counter : Outport  Port=2
  wires:
  Constant/1 -> Comparator1/1
  Counter/1 -> counter/1, Comparator1/2
  Comparator1/1 -> finish/1
  sclr/1 -> Counter/2
  ena/1 -> Counter/1
